simulink model "Ex2"  (R2022b)
settings: Solver=VariableStepAuto  StartTime=0.0  StopTime=0.05  RelTol=1e-3
libraries: commrandsrc3 x1
settings Model: Creator=ASUS  LastModifiedBy=mluser
settings ModelReferenceCC: EnableRefExpFcnMdlSchedulingChecks=on

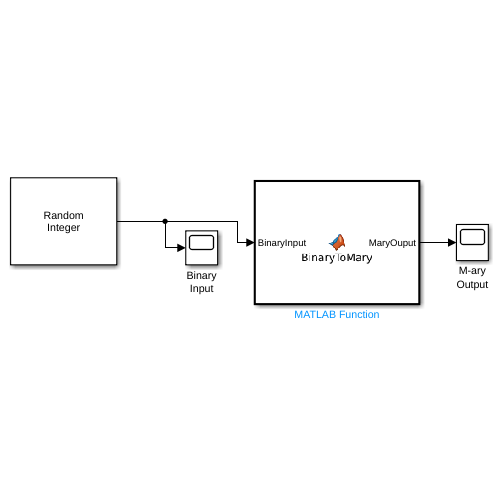
[thumbnail: Simulink's stored preview of the top-level diagram]
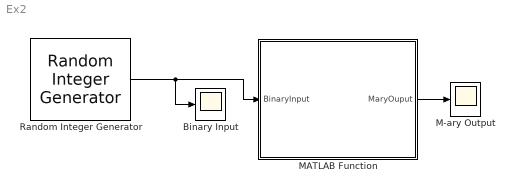
== system Ex2 ==
  Binary Input : Scope
  M-ary Output : Scope
  MATLAB Function : MATLAB Function  TreatAsAtomicUnit=on
  Random Integer Generator : commrandsrc3/Random Integer Generator  SetSize=2  SeedSource=Parameter  Seed=37  SampleTime=1e-3  SamplesPerFrame=1  OutputDataType=double  SimulateUsing=Interpreted execution
  wires:
  MATLAB Function/1(MaryOuput) -> M-ary Output/1
  Random Integer Generator/1 -> Binary Input/1, MATLAB Function/1(BinaryInput)

== matlab function Ex2/MATLAB Function ==
  data: BinaryInput input; MaryOuput output
function MaryOuput = BinaryToMary(BinaryInput)
 persistent v1 v2 v3 vlast flag

 if isempty(flag)
     flag =1;
     v2=0;
     v1=0;
     vlast=0;
 end

 v3=v2;
 v2=v1;
 v1=BinaryInput;

 if (flag==3)
     MaryOuput=4*v3+2*v2+v1;
     vlast=MaryOuput;
     flag=1;
 else
     flag=flag+1;
     MaryOuput=vlast;
 end
